simulink subsystem "balloon_drag"  (R2020a)
settings: Solver=VariableStepAuto  StartTime=0.0  StopTime=10.0  RelTol=1e-3
settings Model: Creator=Philip  LastModifiedBy=Philip

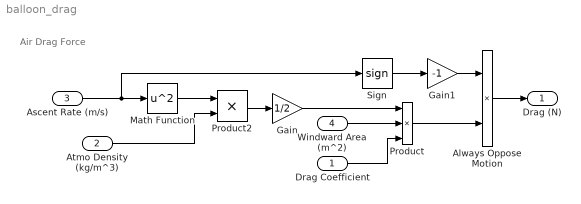
== system balloon_drag ==
  note: Air Drag Force
  Drag Coefficient : Inport
  Atmo Density (kg/m^3) : Inport  Port=2
  Ascent Rate (m/s) : Inport  Port=3
  Windward Area (m^2) : Inport  Port=4
  Always Oppose Motion : Product
  Gain : Gain  Gain=1/2
  Gain1 : Gain  Gain=-1
  Math Function : Math  Operator=square  SaturateOnIntegerOverflow=on
  Product : Product  Inputs=3
  Product2 : Product
  Sign : Signum
  Drag (N) : Outport
  wires:
  Atmo Density (kg/m^3)/1 -> Product2/2
  Ascent Rate (m/s)/1 -> Math Function/1, Sign/1
  Math Function/1 -> Product2/1
  Product2/1 -> Gain/1
  Product/1 -> Always Oppose Motion/2
  Windward Area (m^2)/1 -> Product/2
  Drag Coefficient/1 -> Product/3
  Gain/1 -> Product/1
  Always Oppose Motion/1 -> Drag (N)/1
  Gain1/1 -> Always Oppose Motion/1
  Sign/1 -> Gain1/1
